simulink model "WMC_Ver_03_Final_Model"  (R2026a)
settings: Solver=FixedStepAuto  StopTime=inf  FixedStep=0.1
settings Model: PacingRate=5  Creator=Rakshith  LastModifiedBy=Rakshith

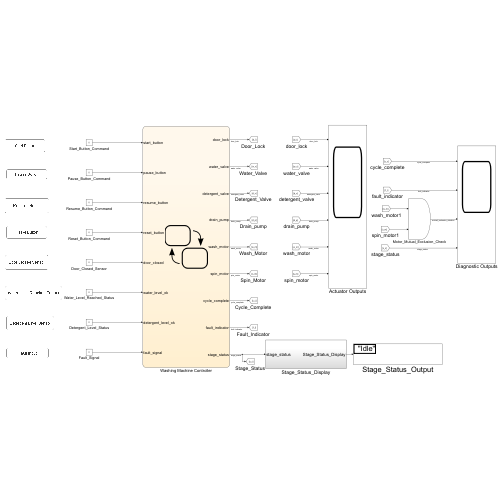
[thumbnail: Simulink's stored preview of the top-level diagram]
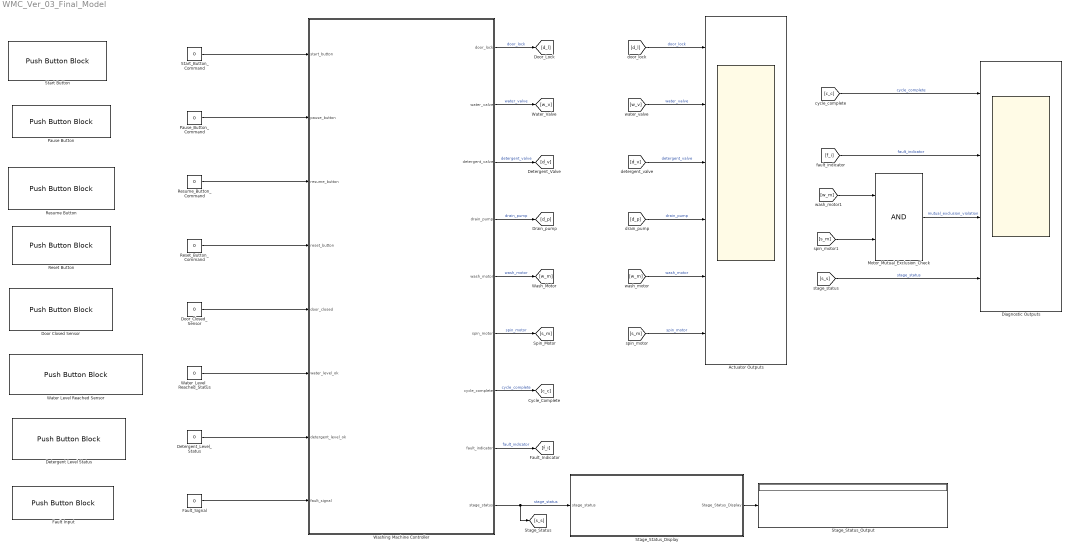
== system WMC_Ver_03_Final_Model ==
  Actuator Outputs : Scope  NumInputPorts=6
      settings: ActiveDisplayYMinimum=-0.12499999999999997  ActiveDisplayYMaximum=1.125
  Detergent Level Status : PushButtonBlock  ButtonText=Detergent Level Sensor  ButtonType=Latch  IconOnColor=[0.0, 0.39215686274509803, 0.0]  IconOffColor=[0.0, 1.0, 0.0]  OffValue=0.000000
  Detergent_Level_Status : Constant  Value=0
  Diagnostic Outputs : Scope  NumInputPorts=4
      settings: ActiveDisplayYMinimum=-1  ActiveDisplayYMaximum=1
  Door Closed Sensor : PushButtonBlock  ButtonText=Door Closed Sensor  ButtonType=Latch  IconOnColor=[0.0, 0.39215686274509803, 0.0]  IconOffColor=[0.0, 1.0, 0.0]  OffValue=0.000000
  Door_Closed_Sensor : Constant  Value=0
  Fault Input : PushButtonBlock  ButtonText=Fault Input  ButtonType=Latch  IconOnColor=[0.0, 0.39215686274509803, 0.0]  IconOffColor=[0.0, 1.0, 0.0]  OffValue=0.000000
  Fault_Signal : Constant  Value=0
  Motor_Mutual_Exclusion_Check : Logic  IconShape=distinctive  AllPortsSameDT=off  OutDataTypeStr=boolean
  Pause Button : PushButtonBlock  ButtonText=Pause Button  ButtonType=Latch  IconOnColor=[0.0, 0.39215686274509803, 0.0]  IconOffColor=[0.0, 1.0, 0.0]  OffValue=0.000000
  Pause_Button_Command : Constant  Value=0
  Reset Button : PushButtonBlock  ButtonText=Reset Button  ButtonType=Latch  IconOnColor=[0.0, 0.39215686274509803, 0.0]  IconOffColor=[0.0, 1.0, 0.0]  OffValue=0.000000
  Reset_Button_Command : Constant  Value=0
  Resume Button : PushButtonBlock  ButtonText=Resume Button  ButtonType=Latch  IconOnColor=[0.0, 0.39215686274509803, 0.0]  IconOffColor=[0.0, 1.0, 0.0]  OffValue=0.000000
  Resume_Button_Command : Constant  Value=0
  Stage_Status_Display : Subsystem
  Stage_Status_Output : Display
  Start Button : PushButtonBlock  ButtonText=Start Button  ButtonType=Latch  IconOnColor=[0.0, 0.39215686274509803, 0.0]  IconOffColor=[0.0, 1.0, 0.0]  OffValue=0.000000
  Start_Button_Command : Constant  Value=0
  Washing Machine Controller : Stateflow chart  TreatAsAtomicUnit=on
  Water Level Reached Sensor : PushButtonBlock  ButtonText=Water Level Reached Sensor  ButtonType=Latch  IconOnColor=[0.0, 0.39215686274509803, 0.0]  IconOffColor=[0.0, 1.0, 0.0]  OffValue=0.000000
  Water_Level_Reached_Status : Constant  Value=0
  wires:
  Start_Button_Command/1 -> Washing Machine Controller/1(start_button)
  Pause_Button_Command/1 -> Washing Machine Controller/2(pause_button)
  Resume_Button_Command/1 -> Washing Machine Controller/3(resume_button)
  Reset_Button_Command/1 -> Washing Machine Controller/4(reset_button)
  Door_Closed_Sensor/1 -> Washing Machine Controller/5(door_closed)
  Water_Level_Reached_Status/1 -> Washing Machine Controller/6(water_level_ok)
  Fault_Signal/1 -> Washing Machine Controller/8(fault_signal)
  Detergent_Level_Status/1 -> Washing Machine Controller/7(detergent_level_ok)
  Motor_Mutual_Exclusion_Check/1 -> Diagnostic Outputs/3  "mutual_exclusion_violation"
  Stage_Status_Display/1(Stage_Status_Display) -> Stage_Status_Output/1
  Washing Machine Controller/9(stage_status) -> Stage_Status_Display/1(stage_status), [s_s]  "stage_status"
  Washing Machine Controller/1(door_lock) -> [d_l]  "door_lock"
  [d_l] -> Actuator Outputs/1  "door_lock"
  Washing Machine Controller/2(water_valve) -> [w_v]  "water_valve"
  [w_v] -> Actuator Outputs/2  "water_valve"
  Washing Machine Controller/3(detergent_valve) -> [d_v]  "detergent_valve"
  [d_v] -> Actuator Outputs/3  "detergent_valve"
  Washing Machine Controller/4(drain_pump) -> [d_p]  "drain_pump"
  [d_p] -> Actuator Outputs/4  "drain_pump"
  Washing Machine Controller/5(wash_motor) -> [w_m]  "wash_motor"
  [w_m] -> Actuator Outputs/5  "wash_motor"
  Washing Machine Controller/6(spin_motor) -> [s_m]  "spin_motor"
  [s_m] -> Actuator Outputs/6  "spin_motor"
  [s_m] -> Motor_Mutual_Exclusion_Check/2
  [w_m] -> Motor_Mutual_Exclusion_Check/1
  Washing Machine Controller/7(cycle_complete) -> [c_c]  "cycle_complete"
  [c_c] -> Diagnostic Outputs/1  "cycle_complete"
  Washing Machine Controller/8(fault_indicator) -> [f_i]  "fault_indicator"
  [f_i] -> Diagnostic Outputs/2  "fault_indicator"
  [s_s] -> Diagnostic Outputs/4  "stage_status"

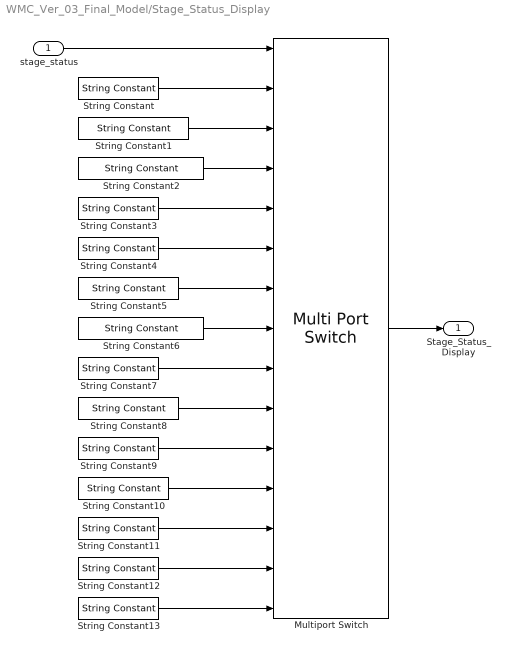
== system WMC_Ver_03_Final_Model/Stage_Status_Display ==
  stage_status : Inport
  Multiport Switch : MultiPortSwitch  DataPortOrder=Zero-based contiguous  Inputs=13  DataPortForDefault=Additional data port  zeroidx=on  SaturateOnIntegerOverflow=off  InputSameDT=off
  String Constant : StringConstant  String="\"Idle\""
  String Constant1 : StringConstant  String="\"Door_Lock_Activation\""
  String Constant10 : StringConstant  String="\"Cycle_Complete\""
  String Constant11 : StringConstant  String="\"Paused\""
  String Constant12 : StringConstant  String="\"Fault\""
  String Constant13 : StringConstant  String="\"Invalid_Status\""
  String Constant2 : StringConstant  String="\"Water_Fill_Wash_Cycle\""
  String Constant3 : StringConstant  String="\"Detergent_Fill\""
  String Constant4 : StringConstant  String="\"Wash\""
  String Constant5 : StringConstant  String="\"Drain_Wash_Cycle\""
  String Constant6 : StringConstant  String="\"Water_Fill_Rinse_Cycle\""
  String Constant7 : StringConstant  String="\"Rinse\""
  String Constant8 : StringConstant  String="\"Drain_Rinse_Cycle\""
  String Constant9 : StringConstant  String="\"Spin\""
  Stage_Status_Display : Outport
  wires:
  String Constant2/1 -> Multiport Switch/4
  String Constant/1 -> Multiport Switch/2
  stage_status/1 -> Multiport Switch/1
  String Constant1/1 -> Multiport Switch/3
  Multiport Switch/1 -> Stage_Status_Display/1
  String Constant3/1 -> Multiport Switch/5
  String Constant4/1 -> Multiport Switch/6
  String Constant5/1 -> Multiport Switch/7
  String Constant6/1 -> Multiport Switch/8
  String Constant7/1 -> Multiport Switch/9
  String Constant8/1 -> Multiport Switch/10
  String Constant9/1 -> Multiport Switch/11
  String Constant10/1 -> Multiport Switch/12
  String Constant11/1 -> Multiport Switch/13
  String Constant12/1 -> Multiport Switch/14
  String Constant13/1 -> Multiport Switch/15

== stateflow chart WMC_Ver_03_Final_Model/Washing Machine Controller ==
  state Idle
    en: door_lock = 0;
    water_valve = 0;
    detergent_valve = 0;
    drain_pump = 0;
    wash_motor = 0;
    spin_motor = 0;
    cycle_complete = 0;
    fault_indicator = 0;
    stage_status = 0;
  state Active_Washing_Cycle
    (history)
    state Wash
      en: door_lock = 1;
      water_valve = 0;
      detergent_valve = 0;
      drain_pump = 0;
      wash_motor = 1;
      spin_motor = 0;
      cycle_complete = 0;
      stage_status = 4;
    state Water_Fill_Wash_Cycle
      en: door_lock = 1;
      water_valve = 1;
      detergent_valve = 0;
      drain_pump = 0;
      wash_motor = 0;
      spin_motor = 0;
      cycle_complete = 0;
      stage_status = 2;
    state Detergent_Fill
      en: door_lock = 1;
      water_valve = 0;
      detergent_valve = 1;
      drain_pump = 0;
      wash_motor = 0;
      spin_motor = 0;
      cycle_complete = 0;
      stage_status = 3;
    state Rinse
      en: door_lock = 1;
      water_valve = 0;
      detergent_valve = 0;
      drain_pump = 0;
      wash_motor = 1;
      spin_motor = 0;
      cycle_complete = 0;
      stage_status = 7;
    state Drain_Wash_Cycle
      en: door_lock = 1;
      water_valve = 0;
      detergent_valve = 0;
      drain_pump = 1;
      wash_motor = 0;
      spin_motor = 0;
      cycle_complete = 0;
      stage_status = 5;
    state Water_Fill_Rinse_Cycle
      en: door_lock = 1;
      water_valve = 1;
      detergent_valve = 0;
      drain_pump = 0;
      wash_motor = 0;
      spin_motor = 0;
      cycle_complete = 0;
      stage_status = 6;
    state Spin
      en: door_lock = 1;
      water_valve = 0;
      detergent_valve = 0;
      drain_pump = 0;
      wash_motor = 0;
      spin_motor = 1;
      cycle_complete = 0;
      stage_status = 9;
    state Cycle_Complete
      en: door_lock = 0;
      water_valve = 0;
      detergent_valve = 0;
      drain_pump = 0;
      wash_motor = 0;
      spin_motor = 0;
      cycle_complete = 1;
      stage_status = 10;
    state Drain_Rinse_Cycle
      en: door_lock = 1;
      water_valve = 0;
      detergent_valve = 0;
      drain_pump = 1;
      wash_motor = 0;
      spin_motor = 0;
      cycle_complete = 0;
      stage_status = 8;
    (default) -> Water_Fill_Wash_Cycle
    Water_Fill_Wash_Cycle -> Detergent_Fill : [water_level_ok == 1]
    Detergent_Fill -> Wash [order 1] : [detergent_level_ok == 1]
    Wash -> Drain_Wash_Cycle : [after(wash_duration, sec)]
    Water_Fill_Rinse_Cycle -> Rinse : [water_level_ok == 1]
    Drain_Wash_Cycle -> Water_Fill_Rinse_Cycle : [after(drain_duration, sec)]
    Rinse -> Drain_Rinse_Cycle : [after(rinse_duration, sec)]
    Drain_Rinse_Cycle -> Spin : [after(drain_duration, sec)]
    Spin -> Cycle_Complete : [after(spin_duration, sec)]
  state Door_Lock_Activation
    en: door_lock = 1;
    water_valve = 0;
    detergent_valve = 0;
    drain_pump = 0;
    wash_motor = 0;
    spin_motor = 0;
    cycle_complete = 0;
    stage_status = 1;
  state Paused
    en: door_lock = 1;
    water_valve = 0;
    detergent_valve = 0;
    drain_pump = 0;
    wash_motor = 0;
    spin_motor = 0;
    cycle_complete = 0;
    stage_status = 11;
  state Fault
    en:  door_lock = 1;
    water_valve = 0;
    detergent_valve = 0;
    drain_pump = 0;
    wash_motor = 0;
    spin_motor = 0;
    cycle_complete = 0;
    fault_indicator =  1;
    stage_status = 12;
  (default) -> Idle
  Cycle_Complete -> Idle : [after(10, sec)]
  Fault -> Idle : [reset_button == 1 & fault_signal == 0]
  Door_Lock_Activation -> Idle [order 1] : [door_closed == 0]
  Idle -> Door_Lock_Activation : [start_button == 1 && door_closed == 1]
  Door_Lock_Activation -> Water_Fill_Wash_Cycle [order 2] : [after(door_lock_delay, sec) && door_closed == 1]
  Detergent_Fill -> Fault [order 2] : [after(detergent_fill_timeout, sec) && detergent_level_ok == 0]
  Active_Washing_Cycle -> Paused [order 2] : [pause_button == 1]
  Paused -> Active_Washing_Cycle : [resume_button && door_closed == 1]
  Active_Washing_Cycle -> Fault [order 1] : [fault_signal == 1]
  data: door_lock output; water_valve output; start_button input; pause_button input; resume_button input; reset_button input; door_closed input; water_level_ok input; detergent_level_ok input; detergent_valve output; drain_pump output; wash_motor output; spin_motor output; cycle_complete output; fault_indicator output; wash_duration local =20*60; drain_duration local =4*60; rinse_duration local =15*60; spin_duration local =10*60; door_lock_delay local =10; fault_signal input; detergent_fill_timeout local =30; stage_status output
